simulink model "momentum_dump_test_rev2"  (R2016b)
settings: Solver=VariableStepAuto  StartTime=0.0  StopTime=2500  MinStep=0.001  RelTol=1e-3
values from neighbouring files (symbols this model uses):
  fsw_params = init_fsw_params()    [momentum_unload_test_init.m]
undefined symbols (not defined in the file or in its folder): body_rates_radps, command_processing, DiscIntNeverNeededParam, disturbances_lib, DT_aero_eci_Nm, DT_dipole_body_Am2, DT_grav_eci_Nm, DT_solar_eci_Nm, env_acc_eci_mps2, Environment, environment_lib, GPS_time, init_pos_eci_km, init_vel_eci_kmps, mag_vec_eci, magnetorquer_assembly_lib, position_eci_km, quaternion, RW_assembly_simple_lib, sim_params, sun_vec_eci, velocity_eci_kmps
libraries: aerolibutil x10, simulink x6, bus_stubs_template x3, aerolibactuator x3, vrlib x2, dynamics_lib x1, GPS_time_lib x1, aero_drag_lib x1, gravity_lib_2 x1, mag_vec_lib x1, solar_pressure_lib x1, sun_vector_lib x1
settings Model: Creator=evich  LastModifiedBy=evich

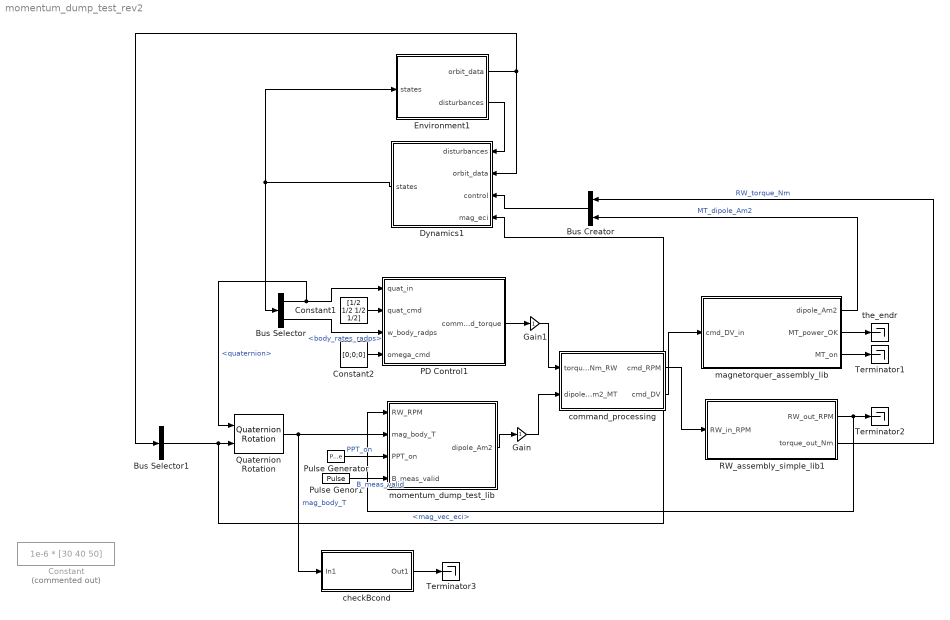
== system momentum_dump_test_rev2 ==
  Bus Creator : BusCreator  Inputs=2
  Bus Selector : BusSelector  OutputSignals=quaternion,body_rates_radps
  Bus Selector1 : BusSelector  OutputSignals=mag_vec_eci
  Constant : Constant  Commented=on  Value=1e-6 * [30 40 50]
  Constant1 : Constant  Value=[1/2 1/2 1/2 1/2]
  Constant2 : Constant  Value=[0;0;0]
  Dynamics1 : Subsystem  AncestorBlock=dynamics_lib/Dynamics
  Environment1 : Subsystem  AncestorBlock=environment_lib/Environment
  Gain : Gain
  Gain1 : Gain
  PD Control1 : Subsystem  AncestorBlock=pd_control_lib/PD Control
  Pulse Generator : DiscretePulseGenerator  PulseType=Time based  Period=fsw_params.actuators.ppt.sync_pulse  PulseWidth=fsw_params.actuators.ppt.t_charge_pct
  Pulse Genor1 : DiscretePulseGenerator  PulseType=Time based  Period=10  PulseWidth=sim_params.sensors.magnetometer.valid_pct
  Quaternion Rotation : aerolibutil/Quaternion Rotation
  RW_assembly_simple_lib1 : Subsystem  AncestorBlock=RW_assembly_simple_lib/RW_assembly_simple_lib  mask{natural_frequency=sim_params.actuators.reaction_wheel.natural_freq, damping_ratio=sim_params.actuators.reaction_wheel.damping, max_rate=sim_params.actuators.reaction_wheel.rate_limit}
      mask prompts: natural_frequency "aeroblks:aeroblkactuator:blockNonlinearSecondOrderActuatorParamNaturalfrequency"; damping_ratio "aeroblks:aeroblkactuator:blockNonlinearSecondOrderActuatorParamDampingratio"; max_rate "aeroblks:aeroblkactuator:blockNonlinearSecondOrderActuatorParamRatelimit"
      mask TypeOptions natural_frequency: Nonlinear Second-Order Actuator/wn_fin | Nonlinear Second-Order Actuator1/wn_fin | Nonlinear Second-Order Actuator2/wn_fin
      mask TypeOptions damping_ratio: Nonlinear Second-Order Actuator/z_fin | Nonlinear Second-Order Actuator1/z_fin | Nonlinear Second-Order Actuator2/z_fin
      mask TypeOptions max_rate: Nonlinear Second-Order Actuator/fin_maxrate | Nonlinear Second-Order Actuator1/fin_maxrate | Nonlinear Second-Order Actuator2/fin_maxrate
  Terminator1 : Terminator
  Terminator2 : Terminator
  Terminator3 : Terminator
  checkBcond : Subsystem
  command_processing : Subsystem  AncestorBlock=command_processing/command_processing
  magnetorquer_assembly_lib : Subsystem  AncestorBlock=magnetorquer_assembly_lib/magnetorquer_assembly_lib
  momentum_dump_test_lib : Subsystem
  the_endr : Terminator
  wires:
  Dynamics1/1(states) -> Environment1/1(states), Bus Selector/1
  Environment1/2(disturbances) -> Dynamics1/1(disturbances)
  Environment1/1(orbit_data) -> Bus Selector1/1, Dynamics1/2(orbit_data)
  Bus Creator/1 -> Dynamics1/3(control)
  RW_assembly_simple_lib1/2(torque_out_Nm) -> Bus Creator/1  "RW_torque_Nm"
  magnetorquer_assembly_lib/1(dipole_Am2) -> Bus Creator/2  "MT_dipole_Am2"
  Bus Selector/1 -> PD Control1/1(quat_in), Quaternion Rotation/1  "<quaternion>"
  Bus Selector/2 -> PD Control1/3(w_body_radps)  "<body_rates_radps>"
  command_processing/1(cmd_RPM) -> RW_assembly_simple_lib1/1(RW_in_RPM)
  command_processing/2(cmd_DV) -> magnetorquer_assembly_lib/1(cmd_DV_in)
  PD Control1/1(command_torque) -> Gain1/1
  momentum_dump_test_lib/1(dipole_Am2) -> Gain/1
  Pulse Generator/1 -> momentum_dump_test_lib/3(PPT_on)  "PPT_on"
  Pulse Genor1/1 -> momentum_dump_test_lib/4(B_meas_valid)  "B_meas_valid"
  Constant1/1 -> PD Control1/2(quat_cmd)
  Constant2/1 -> PD Control1/4(omega_cmd)
  magnetorquer_assembly_lib/2(MT_power_OK) -> the_endr/1
  magnetorquer_assembly_lib/3(MT_on) -> Terminator1/1
  RW_assembly_simple_lib1/1(RW_out_RPM) -> momentum_dump_test_lib/1(RW_RPM), Terminator2/1
  Bus Selector1/1 -> Dynamics1/4(mag_eci), Quaternion Rotation/2  "<mag_vec_eci>"
  Quaternion Rotation/1 -> checkBcond/1(In1), momentum_dump_test_lib/2(mag_body_T)  "mag_body_T"
  Gain/1 -> command_processing/2(dipole_Am2_MT)
  Gain1/1 -> command_processing/1(torque_Nm_RW)
  checkBcond/1(Out1) -> Terminator3/1

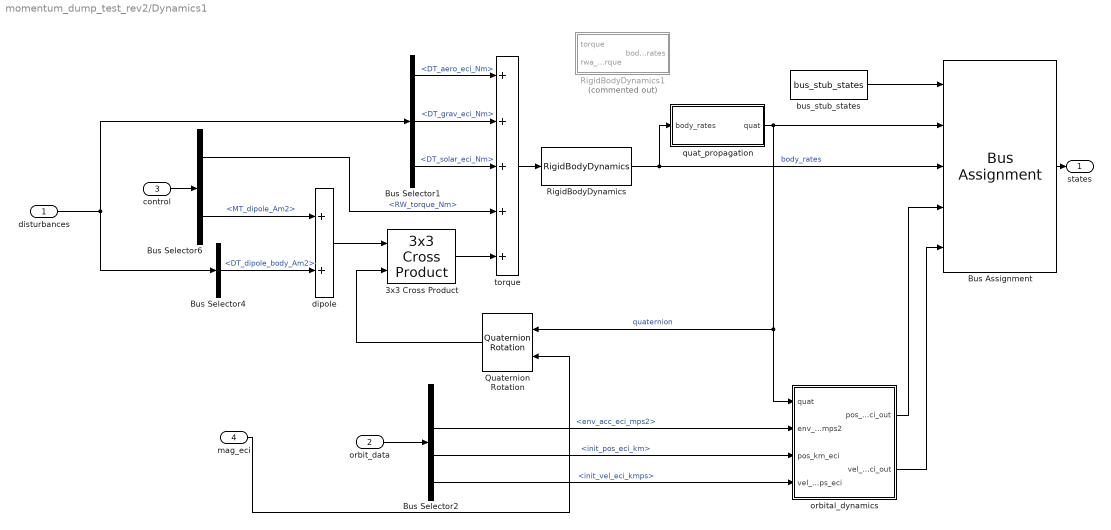
== system momentum_dump_test_rev2/Dynamics1 ==
  disturbances : Inport  OutDataTypeStr=Bus: disturbances
  orbit_data : Inport  Port=2  OutDataTypeStr=Bus: orbit_data
  control : Inport  Port=3  OutDataTypeStr=Bus: control
  mag_eci : Inport  Port=4
  3x3 Cross Product : aerolibutil/3x3 Cross Product
  Bus Assignment : BusAssignment  AssignedSignals=quaternion,body_rates_radps,position_eci_km,velocity_eci_kmps
  Bus Selector1 : BusSelector  OutputSignals=DT_aero_eci_Nm,DT_grav_eci_Nm,DT_solar_eci_Nm
  Bus Selector2 : BusSelector  OutputSignals=mag_vec_eci,env_acc_eci_mps2,init_pos_eci_km,init_vel_eci_kmps
  Bus Selector4 : BusSelector  OutputSignals=DT_dipole_body_Am2
  Bus Selector6 : BusSelector  OutputSignals=RW_torque_Nm,MT_dipole_Am2
  Quaternion Rotation : aerolibutil/Quaternion Rotation
  RigidBodyDynamics : dynamics_lib/Dynamics/RigidBodyDynamics
  RigidBodyDynamics1 : Subsystem  Commented=on
  bus_stub_states : bus_stubs_template/bus_stub_states
  dipole : Sum  Inputs=2
  orbital_dynamics : Subsystem
  quat_propagation : Subsystem
  torque : Sum  Inputs=5
  states : Outport
  wires:
  Bus Assignment/1 -> states/1
  bus_stub_states/1 -> Bus Assignment/1
  quat_propagation/1(quat) -> Bus Assignment/2, Quaternion Rotation/1, orbital_dynamics/1(quat)  "quaternion"
  RigidBodyDynamics/1 -> quat_propagation/1(body_rates), Bus Assignment/3  "body_rates"
  disturbances/1 -> Bus Selector4/1, Bus Selector1/1
  Bus Selector1/1 -> torque/1  "<DT_aero_eci_Nm>"
  Bus Selector1/2 -> torque/2  "<DT_grav_eci_Nm>"
  Bus Selector1/3 -> torque/3  "<DT_solar_eci_Nm>"
  control/1 -> Bus Selector6/1
  Bus Selector6/1 -> torque/4  "<RW_torque_Nm>"
  Bus Selector4/1 -> dipole/2  "<DT_dipole_body_Am2>"
  Bus Selector6/2 -> dipole/1  "<MT_dipole_Am2>"
  torque/1 -> RigidBodyDynamics/1
  dipole/1 -> 3x3 Cross Product/1
  Quaternion Rotation/1 -> 3x3 Cross Product/2
  3x3 Cross Product/1 -> torque/5
  Bus Selector2/2 -> orbital_dynamics/2(env_accel_eci_mps2)  "<env_acc_eci_mps2>"
  mag_eci/1 -> Quaternion Rotation/2
  orbital_dynamics/2(vel_kmps_eci_out) -> Bus Assignment/5
  orbital_dynamics/1(pos_km_eci_out) -> Bus Assignment/4
  Bus Selector2/3 -> orbital_dynamics/3(pos_km_eci)  "<init_pos_eci_km>"
  Bus Selector2/4 -> orbital_dynamics/4(vel_kmps_eci)  "<init_vel_eci_kmps>"
  orbit_data/1 -> Bus Selector2/1

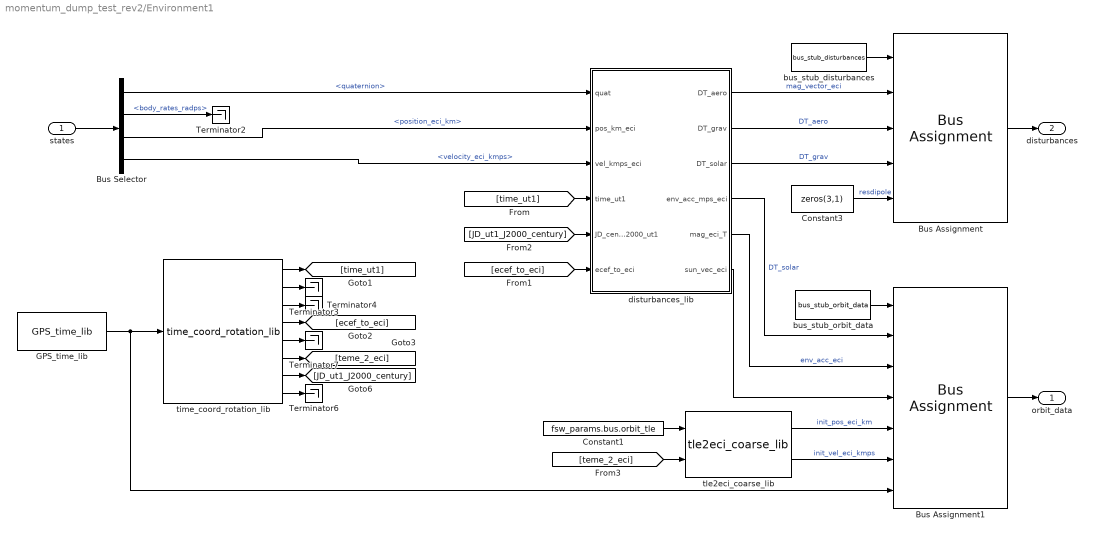
== system momentum_dump_test_rev2/Environment1 ==
  states : Inport  OutDataTypeStr=Bus: states
  Bus Assignment : BusAssignment  AssignedSignals=DT_aero_eci_Nm,DT_grav_eci_Nm,DT_solar_eci_Nm,DT_dipole_body_Am2
  Bus Assignment1 : BusAssignment  AssignedSignals=env_acc_eci_mps2,mag_vec_eci,sun_vec_eci,init_pos_eci_km,init_vel_eci_kmps,GPS_time
  Bus Selector : BusSelector  OutputSignals=quaternion,body_rates_radps,position_eci_km,velocity_eci_kmps
  Constant1 : Constant  Value=fsw_params.bus.orbit_tle
  Constant3 : Constant  Value=zeros(3,1)
  GPS_time_lib : GPS_time_lib/GPS_time_lib
  Terminator{2..4,6..7} (5 alike) : Terminator
  bus_stub_disturbances : bus_stubs_template/bus_stub_disturbances
  bus_stub_orbit_data : bus_stubs_template/bus_stub_orbit_data
  disturbances_lib : Subsystem  AncestorBlock=disturbances_lib/disturbances_lib
  time_coord_rotation_lib : time_coord_rotation_lib/time_coord_rotation_lib
  tle2eci_coarse_lib : tle2eci_coarse_lib/tle2eci_coarse_lib
  orbit_data : Outport
  disturbances : Outport  Port=2
  wires:
  tle2eci_coarse_lib/2 -> Bus Assignment1/6  "init_vel_eci_kmps"
  tle2eci_coarse_lib/1 -> Bus Assignment1/5  "init_pos_eci_km"
  Constant1/1 -> tle2eci_coarse_lib/1
  bus_stub_disturbances/1 -> Bus Assignment/1
  Bus Assignment/1 -> disturbances/1
  states/1 -> Bus Selector/1
  Bus Selector/1 -> disturbances_lib/1(quat)  "<quaternion>"
  Bus Selector/2 -> Terminator2/1  "<body_rates_radps>"
  Bus Selector/3 -> disturbances_lib/2(pos_km_eci)  "<position_eci_km>"
  Bus Selector/4 -> disturbances_lib/3(vel_kmps_eci)  "<velocity_eci_kmps>"
  [time_ut1] -> disturbances_lib/4(time_ut1)
  Constant3/1 -> Bus Assignment/5  "resdipole"
  bus_stub_orbit_data/1 -> Bus Assignment1/1
  Bus Assignment1/1 -> orbit_data/1
  disturbances_lib/6(sun_vec_eci) -> Bus Assignment1/4
  time_coord_rotation_lib/1 -> [time_ut1]
  time_coord_rotation_lib/7 -> [JD_ut1_J2000_century]
  time_coord_rotation_lib/2 -> Terminator3/1
  time_coord_rotation_lib/4 -> [ecef_to_eci]
  [JD_ut1_J2000_century] -> disturbances_lib/5(JD_cent_J2000_ut1)
  [ecef_to_eci] -> disturbances_lib/6(ecef_to_eci)
  disturbances_lib/1(DT_aero) -> Bus Assignment/2  "mag_vector_eci"
  disturbances_lib/2(DT_grav) -> Bus Assignment/3  "DT_aero"
  disturbances_lib/3(DT_solar) -> Bus Assignment/4  "DT_grav"
  disturbances_lib/4(env_acc_mps_eci) -> Bus Assignment1/2  "DT_solar"
  disturbances_lib/5(mag_eci_T) -> Bus Assignment1/3  "env_acc_eci"
  GPS_time_lib/1 -> Bus Assignment1/7, time_coord_rotation_lib/1
  time_coord_rotation_lib/3 -> Terminator4/1
  time_coord_rotation_lib/6 -> [teme_2_eci]
  time_coord_rotation_lib/8 -> Terminator6/1
  time_coord_rotation_lib/5 -> Terminator7/1
  [teme_2_eci] -> tle2eci_coarse_lib/2

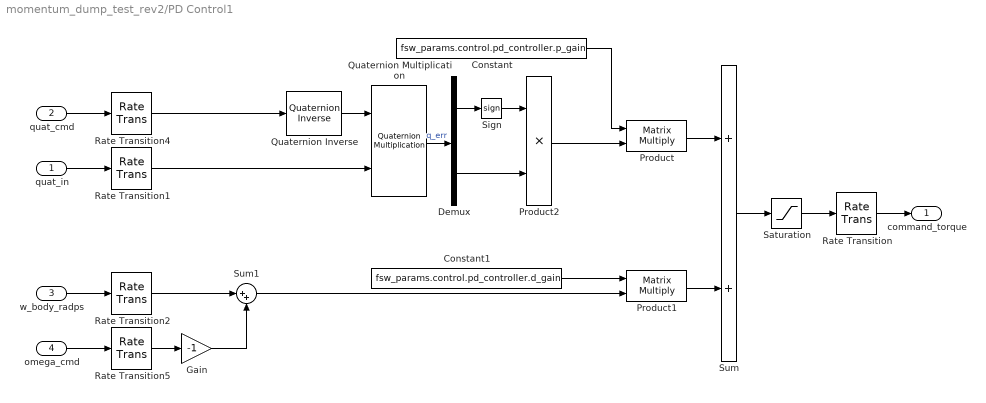
== system momentum_dump_test_rev2/PD Control1 ==
  quat_in : Inport
  quat_cmd : Inport  Port=2
  w_body_radps : Inport  Port=3
  omega_cmd : Inport  Port=4
  Constant : Constant  Value=fsw_params.control.pd_controller.p_gain
  Constant1 : Constant  Value=fsw_params.control.pd_controller.d_gain
  Demux : Demux  Outputs=[1 3]
  Gain : Gain  Gain=-1
  Product : Product  Multiplication=Matrix(*)
  Product1 : Product  Multiplication=Matrix(*)
  Product2 : Product
  Quaternion Inverse : aerolibutil/Quaternion Inverse
  Quaternion Multiplication : aerolibutil/Quaternion Multiplication
  Rate Transition : RateTransition  X0=fsw_params.control.pd_controller.ic.rt_command_torque
  Rate Transition1 : RateTransition  X0=fsw_params.control.pd_controller.ic.rt_quat_in  OutPortSampleTime=fsw_params.control.pd_controller.sample_time_s
  Rate Transition2 : RateTransition  X0=fsw_params.control.pd_controller.ic.rt_w_body_radps  OutPortSampleTime=fsw_params.control.pd_controller.sample_time_s
  Rate Transition4 : RateTransition  X0=fsw_params.control.pd_controller.ic.rt_quat_in  OutPortSampleTime=fsw_params.control.pd_controller.sample_time_s
  Rate Transition5 : RateTransition  X0=fsw_params.control.pd_controller.ic.rt_w_body_radps  OutPortSampleTime=fsw_params.control.pd_controller.sample_time_s
  Saturation : Saturate  UpperLimit=fsw_params.control.pd_controller.max_torque  LowerLimit=-fsw_params.control.pd_controller.max_torque
  Sign : Signum
  Sum : Sum
  Sum1 : Sum  Inputs=|++
  command_torque : Outport
  wires:
  Saturation/1 -> Rate Transition/1
  Constant1/1 -> Product1/1
  Constant/1 -> Product/1
  quat_cmd/1 -> Rate Transition4/1
  Quaternion Inverse/1 -> Quaternion Multiplication/1
  quat_in/1 -> Rate Transition1/1
  Quaternion Multiplication/1 -> Demux/1  "q_err"
  Demux/1 -> Sign/1
  w_body_radps/1 -> Rate Transition2/1
  Demux/2 -> Product2/2
  Product/1 -> Sum/1
  Product1/1 -> Sum/2
  Sum/1 -> Saturation/1
  Rate Transition/1 -> command_torque/1
  Rate Transition1/1 -> Quaternion Multiplication/2
  Rate Transition4/1 -> Quaternion Inverse/1
  omega_cmd/1 -> Rate Transition5/1
  Rate Transition2/1 -> Sum1/1
  Rate Transition5/1 -> Gain/1
  Gain/1 -> Sum1/2
  Sum1/1 -> Product1/2
  Sign/1 -> Product2/1
  Product2/1 -> Product/2

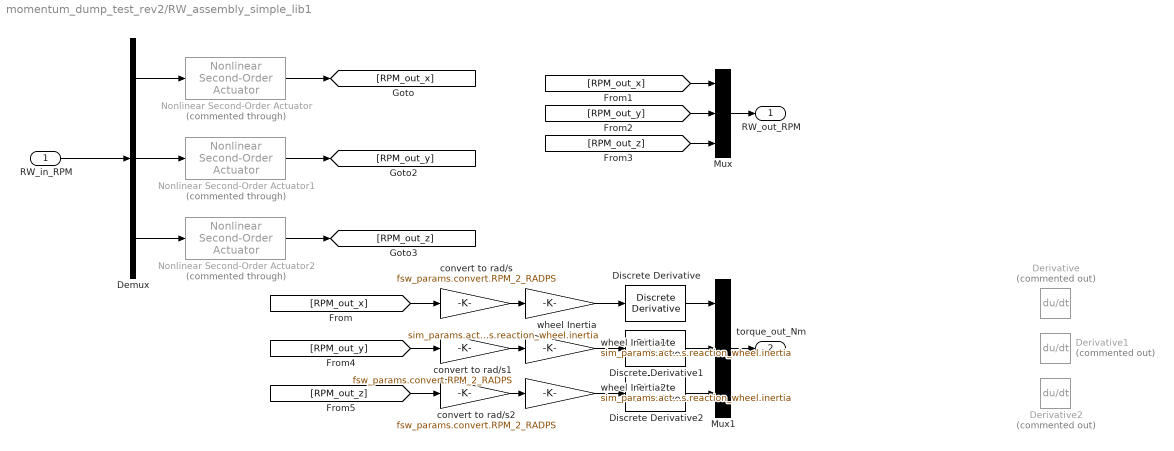
== system momentum_dump_test_rev2/RW_assembly_simple_lib1 ==
  RW_in_RPM : Inport
  Demux : Demux  Outputs=3
  Derivative : Derivative  Commented=on
  Derivative1 : Derivative  Commented=on
  Derivative2 : Derivative  Commented=on
  Discrete Derivative : simulink/Discrete/Discrete Derivative  gainval=1.0  ICPrevScaledInput=sim_params.actuators.reaction_wheel.ic.deriv1  OutMin=[]  OutMax=[]  OutDataType=fixdt(1, 16)  OutScaling=2^-10  DoSatur=off
  Discrete Derivative1 : simulink/Discrete/Discrete Derivative  gainval=1.0  ICPrevScaledInput=sim_params.actuators.reaction_wheel.ic.deriv1  OutMin=[]  OutMax=[]  OutDataType=fixdt(1, 16)  OutScaling=2^-10  DoSatur=off
  Discrete Derivative2 : simulink/Discrete/Discrete Derivative  gainval=1.0  ICPrevScaledInput=sim_params.actuators.reaction_wheel.ic.deriv1  OutMin=[]  OutMax=[]  OutDataType=fixdt(1, 16)  OutScaling=2^-10  DoSatur=off
  Mux : Mux  Inputs=3
  Mux1 : Mux  Inputs=3
  Nonlinear Second-Order Actuator : aerolibactuator/Nonlinear Second-Order Actuator  Commented=through  wn_fin=natural_frequency  z_fin=damping_ratio  fin_max=inf  fin_min=-inf  fin_maxrate=max_rate  fin_act_0=0  fin_act_vel=0
  Nonlinear Second-Order Actuator1 : aerolibactuator/Nonlinear Second-Order Actuator  Commented=through  wn_fin=natural_frequency  z_fin=damping_ratio  fin_max=inf  fin_min=-inf  fin_maxrate=max_rate  fin_act_0=0  fin_act_vel=0
  Nonlinear Second-Order Actuator2 : aerolibactuator/Nonlinear Second-Order Actuator  Commented=through  wn_fin=natural_frequency  z_fin=damping_ratio  fin_max=inf  fin_min=-inf  fin_maxrate=max_rate  fin_act_0=0  fin_act_vel=0
  convert to rad/s : Gain  Gain=fsw_params.convert.RPM_2_RADPS
  convert to rad/s1 : Gain  Gain=fsw_params.convert.RPM_2_RADPS
  convert to rad/s2 : Gain  Gain=fsw_params.convert.RPM_2_RADPS
  wheel Inertia : Gain  Gain=sim_params.actuators.reaction_wheel.inertia
  wheel Inertia1 : Gain  Gain=sim_params.actuators.reaction_wheel.inertia
  wheel Inertia2 : Gain  Gain=sim_params.actuators.reaction_wheel.inertia
  RW_out_RPM : Outport
  torque_out_Nm : Outport  Port=2
  wires:
  RW_in_RPM/1 -> Demux/1
  Demux/1 -> Nonlinear Second-Order Actuator/1
  Demux/2 -> Nonlinear Second-Order Actuator1/1
  Demux/3 -> Nonlinear Second-Order Actuator2/1
  Nonlinear Second-Order Actuator/1 -> [RPM_out_x]
  convert to rad/s/1 -> wheel Inertia/1
  Nonlinear Second-Order Actuator1/1 -> [RPM_out_y]
  Nonlinear Second-Order Actuator2/1 -> [RPM_out_z]
  [RPM_out_x] -> convert to rad/s/1
  [RPM_out_x] -> Mux/1
  [RPM_out_y] -> Mux/2
  [RPM_out_z] -> Mux/3
  Mux/1 -> RW_out_RPM/1
  convert to rad/s1/1 -> wheel Inertia1/1
  [RPM_out_y] -> convert to rad/s1/1
  convert to rad/s2/1 -> wheel Inertia2/1
  [RPM_out_z] -> convert to rad/s2/1
  Mux1/1 -> torque_out_Nm/1
  Discrete Derivative/1 -> Mux1/1
  wheel Inertia/1 -> Discrete Derivative/1
  Discrete Derivative1/1 -> Mux1/2
  Discrete Derivative2/1 -> Mux1/3
  wheel Inertia2/1 -> Discrete Derivative2/1
  wheel Inertia1/1 -> Discrete Derivative1/1

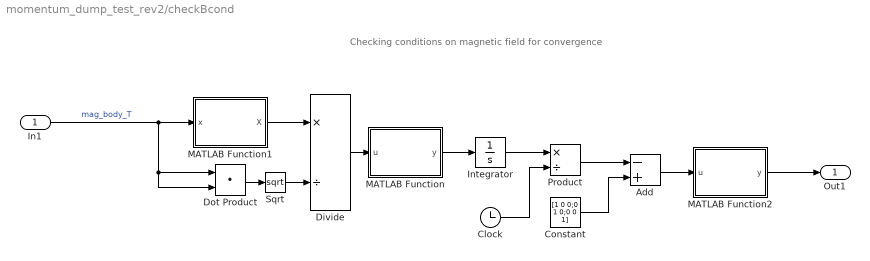
== system momentum_dump_test_rev2/checkBcond ==
  note: Checking conditions on magnetic field for convergence
  In1 : Inport
  Add : Sum  Inputs=-+
  Clock : Clock
      settings: Decimation=10000
  Constant : Constant  Value=[1 0 0;0 1 0;0 0 1]
  Divide : Product  Inputs=*/
  Dot Product : DotProduct  InputSameDT=on  OutDataTypeStr=Inherit: Inherit via internal rule
  Integrator : Integrator  InitialCondition=fsw_params.control.p_dump.ic.delay_B*fsw_params.control.p_dump.ic.delay_B'
  MATLAB Function : MATLAB Function  TreatAsAtomicUnit=on
  MATLAB Function1 : MATLAB Function  TreatAsAtomicUnit=on
  MATLAB Function2 : MATLAB Function  TreatAsAtomicUnit=on
  Product : Product  Inputs=*/
  Sqrt : Sqrt  SaturateOnIntegerOverflow=on
  Out1 : Outport
  wires:
  In1/1 -> Dot Product/2, Dot Product/1, MATLAB Function1/1(x)  "mag_body_T"
  MATLAB Function/1(y) -> Integrator/1
  Integrator/1 -> Product/1
  Clock/1 -> Product/2
  Dot Product/1 -> Sqrt/1
  MATLAB Function1/1(X) -> Divide/1
  Divide/1 -> MATLAB Function/1(u)
  Sqrt/1 -> Divide/2
  Product/1 -> Add/1
  Constant/1 -> Add/2
  Add/1 -> MATLAB Function2/1(u)
  MATLAB Function2/1(y) -> Out1/1

== system momentum_dump_test_rev2/command_processing ==
  torque_Nm_RW : Inport
  dipole_Am2_MT : Inport  Port=2
  dipole-2-digVal : Subsystem
  torque-2-RPM : Subsystem
  cmd_RPM : Outport
  cmd_DV : Outport  Port=2
  wires:
  torque-2-RPM/1(command_RPM) -> cmd_RPM/1
  torque_Nm_RW/1 -> torque-2-RPM/1(cmd_torque_Nm)
  dipole_Am2_MT/1 -> dipole-2-digVal/1(dipole_Am2)
  dipole-2-digVal/1(DigVal) -> cmd_DV/1

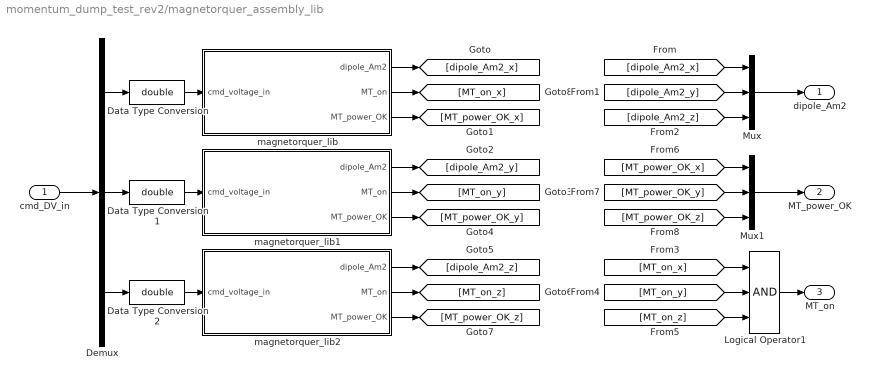
== system momentum_dump_test_rev2/magnetorquer_assembly_lib ==
  cmd_DV_in : Inport
  Data Type Conversion : DataTypeConversion  OutDataTypeStr=double  RndMeth=Nearest
  Data Type Conversion1 : DataTypeConversion  OutDataTypeStr=double  RndMeth=Nearest
  Data Type Conversion2 : DataTypeConversion  OutDataTypeStr=double  RndMeth=Nearest
  Demux : Demux  Outputs=3
  Logical Operator1 : Logic  Inputs=3  AllPortsSameDT=off  OutDataTypeStr=boolean
  Mux : Mux  Inputs=3
  Mux1 : Mux  Inputs=[1 1 1]
  magnetorquer_lib : Subsystem  mask{voltage_to_dipole=fsw_params.control.cmd_processing.dv_2_m_X, upperbound=sim_params.actuators.magnetorquer.max_dipole_x, lowerbound=-sim_params.actuators.magnetorquer.max_dipole_x}
      mask prompts: voltage_to_dipole "Simulink:blkprm_prompts:GainGain"; upperbound "Simulink:masks:UpperBound_MP"; lowerbound "Simulink:masks:LowerBound_MP"
      mask TypeOptions voltage_to_dipole: Gain/Gain
      mask TypeOptions upperbound:
      | Check
      | Static Range/max
      mask TypeOptions lowerbound:
      | Check
      | Static Range/min
  magnetorquer_lib1 : Subsystem  mask{voltage_to_dipole=fsw_params.control.cmd_processing.dv_2_m_Y, upperbound=sim_params.actuators.magnetorquer.max_dipole_y, lowerbound=-sim_params.actuators.magnetorquer.max_dipole_y}
      mask prompts: voltage_to_dipole "Simulink:blkprm_prompts:GainGain"; upperbound "Simulink:masks:UpperBound_MP"; lowerbound "Simulink:masks:LowerBound_MP"
      mask TypeOptions voltage_to_dipole: Gain/Gain
      mask TypeOptions upperbound:
      | Check
      | Static Range/max
      mask TypeOptions lowerbound:
      | Check
      | Static Range/min
  magnetorquer_lib2 : Subsystem  mask{voltage_to_dipole=fsw_params.control.cmd_processing.dv_2_m_Z, upperbound=sim_params.actuators.magnetorquer.max_dipole_z, lowerbound=-sim_params.actuators.magnetorquer.max_dipole_z}
      mask prompts: voltage_to_dipole "Simulink:blkprm_prompts:GainGain"; upperbound "Simulink:masks:UpperBound_MP"; lowerbound "Simulink:masks:LowerBound_MP"
      mask TypeOptions voltage_to_dipole: Gain/Gain
      mask TypeOptions upperbound:
      | Check
      | Static Range/max
      mask TypeOptions lowerbound:
      | Check
      | Static Range/min
  dipole_Am2 : Outport
  MT_power_OK : Outport  Port=2
  MT_on : Outport  Port=3
  wires:
  cmd_DV_in/1 -> Demux/1
  Demux/3 -> Data Type Conversion2/1
  Demux/1 -> Data Type Conversion/1
  Demux/2 -> Data Type Conversion1/1
  magnetorquer_lib/1(dipole_Am2) -> [dipole_Am2_x]
  magnetorquer_lib2/3(MT_power_OK) -> [MT_power_OK_z]
  magnetorquer_lib2/2(MT_on) -> [MT_on_z]
  magnetorquer_lib2/1(dipole_Am2) -> [dipole_Am2_z]
  magnetorquer_lib1/3(MT_power_OK) -> [MT_power_OK_y]
  magnetorquer_lib1/2(MT_on) -> [MT_on_y]
  magnetorquer_lib1/1(dipole_Am2) -> [dipole_Am2_y]
  magnetorquer_lib/3(MT_power_OK) -> [MT_power_OK_x]
  magnetorquer_lib/2(MT_on) -> [MT_on_x]
  Mux/1 -> dipole_Am2/1
  [dipole_Am2_x] -> Mux/1
  [dipole_Am2_y] -> Mux/2
  [dipole_Am2_z] -> Mux/3
  [MT_on_x] -> Logical Operator1/1
  [MT_on_y] -> Logical Operator1/2
  [MT_on_z] -> Logical Operator1/3
  [MT_power_OK_x] -> Mux1/1
  [MT_power_OK_y] -> Mux1/2
  [MT_power_OK_z] -> Mux1/3
  Mux1/1 -> MT_power_OK/1
  Logical Operator1/1 -> MT_on/1
  Data Type Conversion/1 -> magnetorquer_lib/1(cmd_voltage_in)
  Data Type Conversion1/1 -> magnetorquer_lib1/1(cmd_voltage_in)
  Data Type Conversion2/1 -> magnetorquer_lib2/1(cmd_voltage_in)

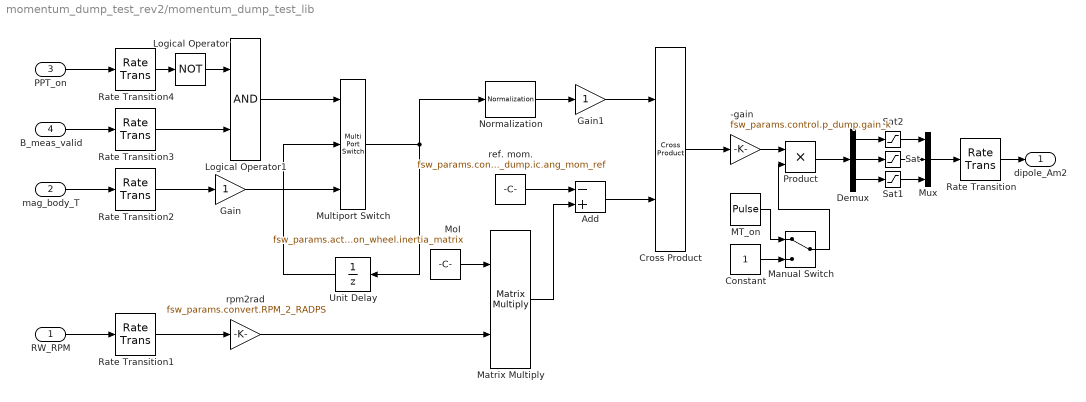
== system momentum_dump_test_rev2/momentum_dump_test_lib ==
  RW_RPM : Inport
  mag_body_T : Inport  Port=2
  PPT_on : Inport  Port=3
  B_meas_valid : Inport  Port=4
  -gain : Gain  Gain=fsw_params.control.p_dump.gain_k
  Add : Sum  Inputs=-+
  Constant : Constant
  Cross Product : vrlib/Utilities/Cross Product
  Demux : Demux  Outputs=3
  Gain : Gain
  Gain1 : Gain
  Logical Operator : Logic  Operator=NOT  AllPortsSameDT=off  OutDataTypeStr=boolean
  Logical Operator1 : Logic  AllPortsSameDT=off  OutDataTypeStr=boolean
  MT_on : DiscretePulseGenerator  PulseType=Time based  Period=1  PulseWidth=fsw_params.actuators.magnetorquer.actuation_time_pct
  Manual Switch : ManualSwitch
  Matrix Multiply : Product  Inputs=**  Multiplication=Matrix(*)
  MoI : Constant  Value=fsw_params.actuators.reaction_wheel.inertia_matrix
  Multiport Switch : MultiPortSwitch  DataPortOrder=Zero-based contiguous  Inputs=2
  Mux : Mux  Inputs=3
  Normalization : dspmathops/Normalization  NormType=Squared 2-norm  Bias=1e-10  NormOver=Each column  Dimension=1  outputDataTypeStr=Inherit: Same as product output  outputLastDataTypeStr=Inherit: Same as product output  outputMin=[]  outputMax=[]  accumDataTypeStr=Inherit: Same as product output  accumLastDataTypeStr=Inherit: Same as product output  roundingMode=Floor  overflowMode=off
  Product : Product
  Rate Transition : RateTransition  X0=fsw_params.control.p_dump.ic.rt_dipole_Am2
  Rate Transition1 : RateTransition  X0=fsw_params.control.p_dump.ic.rt_rw_RPM  OutPortSampleTime=fsw_params.control.p_dump.sample_time_s
  Rate Transition2 : RateTransition  X0=fsw_params.control.p_dump.ic.rt_mag_body_T  OutPortSampleTime=fsw_params.control.p_dump.sample_time_s
  Rate Transition3 : RateTransition  X0=fsw_params.control.p_dump.ic.rt_B_meas_valid  OutPortSampleTime=fsw_params.control.p_dump.sample_time_s
  Rate Transition4 : RateTransition  X0=fsw_params.control.p_dump.ic.rt_PPT_on  OutPortSampleTime=fsw_params.control.p_dump.sample_time_s
  Sat : Saturate  UpperLimit=fsw_params.actuators.magnetorquer.max_dipole_y  LowerLimit=-fsw_params.actuators.magnetorquer.max_dipole_y
  Sat1 : Saturate  UpperLimit=fsw_params.actuators.magnetorquer.max_dipole_z  LowerLimit=-fsw_params.actuators.magnetorquer.max_dipole_z
  Sat2 : Saturate  UpperLimit=fsw_params.actuators.magnetorquer.max_dipole_x  LowerLimit=-fsw_params.actuators.magnetorquer.max_dipole_x
  Unit Delay : UnitDelay  InitialCondition=fsw_params.control.p_dump.ic.rt_mag_body_T  SampleTime=-1
  ref. mom. : Constant  Value=fsw_params.control.p_dump.ic.ang_mom_ref
  rpm2rad : Gain  Gain=fsw_params.convert.RPM_2_RADPS
  dipole_Am2 : Outport
  wires:
  ref. mom./1 -> Add/1
  Matrix Multiply/1 -> Add/2
  MoI/1 -> Matrix Multiply/1
  Multiport Switch/1 -> Normalization/1, Unit Delay/1
  rpm2rad/1 -> Matrix Multiply/2
  Add/1 -> Cross Product/2
  Cross Product/1 -> -gain/1
  Logical Operator1/1 -> Multiport Switch/1
  Logical Operator/1 -> Logical Operator1/1
  Rate Transition3/1 -> Logical Operator1/2
  Rate Transition4/1 -> Logical Operator/1
  Rate Transition2/1 -> Gain/1
  Unit Delay/1 -> Multiport Switch/2
  PPT_on/1 -> Rate Transition4/1
  B_meas_valid/1 -> Rate Transition3/1
  mag_body_T/1 -> Rate Transition2/1
  RW_RPM/1 -> Rate Transition1/1
  Rate Transition1/1 -> rpm2rad/1
  Demux/2 -> Sat/1
  Demux/1 -> Sat2/1
  Demux/3 -> Sat1/1
  Sat1/1 -> Mux/3
  Sat/1 -> Mux/2
  Sat2/1 -> Mux/1
  Mux/1 -> Rate Transition/1
  Gain/1 -> Multiport Switch/3
  Gain1/1 -> Cross Product/1
  Normalization/1 -> Gain1/1
  Rate Transition/1 -> dipole_Am2/1
  -gain/1 -> Product/1
  Product/1 -> Demux/1
  Constant/1 -> Manual Switch/2
  MT_on/1 -> Manual Switch/1
  Manual Switch/1 -> Product/2

== system momentum_dump_test_rev2/Dynamics1/RigidBodyDynamics1 ==
  torque : Inport
  rwa_torque : Inport  Port=2
  Integrator : Integrator  InitialCondition=sim_params.dynamics.ic.rate_init
  Integrator1 : Integrator  InitialCondition=fsw_params.control.cmd_processing.ic.momentum
  dynamics : Subsystem
  body_rates : Outport
  wires:
  dynamics/1(omega_dot) -> Integrator/1
  torque/1 -> dynamics/1(torque)
  Integrator/1 -> dynamics/2(omega), body_rates/1
  rwa_torque/1 -> Integrator1/1
  Integrator1/1 -> dynamics/3(rwa_momentum)

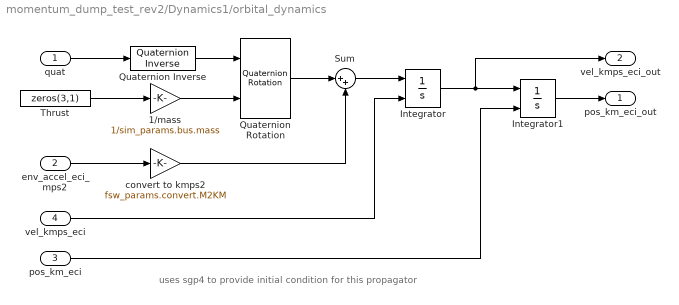
== system momentum_dump_test_rev2/Dynamics1/orbital_dynamics ==
  note: uses sgp4 to provide initial condition for this propagator
  quat : Inport
  env_accel_eci_mps2 : Inport  Port=2
  pos_km_eci : Inport  Port=3
  vel_kmps_eci : Inport  Port=4
  1/mass : Gain  Gain=1/sim_params.bus.mass
  Integrator : Integrator  InitialConditionSource=external  InitialCondition=sim_params.orbit.init_vel_eci
  Integrator1 : Integrator  InitialConditionSource=external  InitialCondition=sim_params.orbit.init_pos_eci
  Quaternion Inverse : aerolibutil/Quaternion Inverse
  Quaternion Rotation : aerolibutil/Quaternion Rotation
  Sum : Sum  Inputs=|++
  Thrust : Constant  Value=zeros(3,1)
  convert to kmps2 : Gain  Gain=fsw_params.convert.M2KM
  pos_km_eci_out : Outport
  vel_kmps_eci_out : Outport  Port=2
  wires:
  convert to kmps2/1 -> Sum/2
  Quaternion Rotation/1 -> Sum/1
  vel_kmps_eci/1 -> Integrator/2
  env_accel_eci_mps2/1 -> convert to kmps2/1
  Integrator/1 -> vel_kmps_eci_out/1, Integrator1/1
  Thrust/1 -> 1/mass/1
  Sum/1 -> Integrator/1
  1/mass/1 -> Quaternion Rotation/2
  Quaternion Inverse/1 -> Quaternion Rotation/1
  pos_km_eci/1 -> Integrator1/2
  quat/1 -> Quaternion Inverse/1
  Integrator1/1 -> pos_km_eci_out/1

== system momentum_dump_test_rev2/Dynamics1/quat_propagation ==
  body_rates : Inport
  Gain1 : Gain  Gain=1/2
  Integrator1 : Integrator  InitialCondition=sim_params.dynamics.ic.quat_init
  MATLAB Function : MATLAB Function  TreatAsAtomicUnit=on
  Product : Product  Multiplication=Matrix(*)  RndMeth=Zero
  Quaternion Normalize : aerolibutil/Quaternion Normalize
  quat : Outport
  wires:
  MATLAB Function/1(Omega) -> Gain1/1
  body_rates/1 -> MATLAB Function/1(w)
  Quaternion Normalize/1 -> Product/2, quat/1
  Gain1/1 -> Product/1
  Integrator1/1 -> Quaternion Normalize/1
  Product/1 -> Integrator1/1

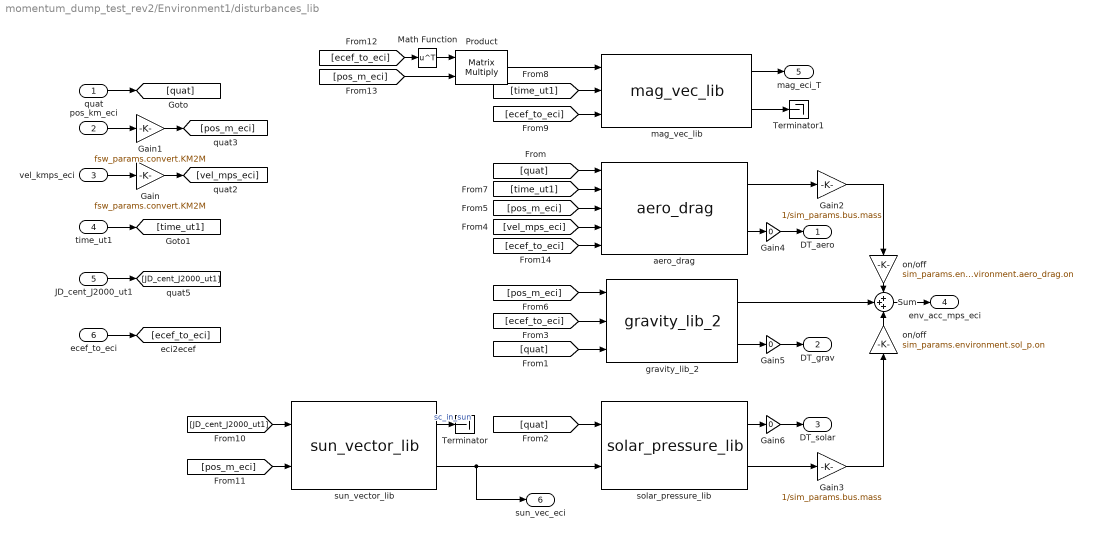
== system momentum_dump_test_rev2/Environment1/disturbances_lib ==
  quat : Inport
  pos_km_eci : Inport  Port=2
  vel_kmps_eci : Inport  Port=3
  time_ut1 : Inport  Port=4
  JD_cent_J2000_ut1 : Inport  Port=5
  ecef_to_eci : Inport  Port=6
  Gain : Gain  Gain=fsw_params.convert.KM2M
  Gain1 : Gain  Gain=fsw_params.convert.KM2M
  Gain2 : Gain  Gain=1/sim_params.bus.mass
  Gain3 : Gain  Gain=1/sim_params.bus.mass
  Gain4 : Gain  Gain=0
  Gain5 : Gain  Gain=0
  Gain6 : Gain  Gain=0
  Math Function : Math  Operator=transpose  SaturateOnIntegerOverflow=on
  Product : Product  Multiplication=Matrix(*)
  Sum : Sum  Inputs=+++
  Terminator : Terminator
  Terminator1 : Terminator
  aero_drag : aero_drag_lib/aero_drag
  gravity_lib_2 : gravity_lib_2/gravity_lib_2
  mag_vec_lib : mag_vec_lib/mag_vec_lib
  on/off : Gain  Gain=sim_params.environment.aero_drag.on
  "on/off " : Gain  Gain=sim_params.environment.sol_p.on
  solar_pressure_lib : solar_pressure_lib/solar_pressure_lib
  sun_vector_lib : sun_vector_lib/sun_vector_lib
  DT_aero : Outport
  DT_grav : Outport  Port=2
  DT_solar : Outport  Port=3
  env_acc_mps_eci : Outport  Port=4
  mag_eci_T : Outport  Port=5
  sun_vec_eci : Outport  Port=6
  wires:
  [ecef_to_eci] -> aero_drag/5
  quat/1 -> [quat]
  ecef_to_eci/1 -> [ecef_to_eci]
  [quat] -> aero_drag/1
  [quat] -> solar_pressure_lib/1
  [ecef_to_eci] -> gravity_lib_2/2
  vel_kmps_eci/1 -> Gain/1
  Gain/1 -> [vel_mps_eci]
  [vel_mps_eci] -> aero_drag/4
  pos_km_eci/1 -> Gain1/1
  Gain1/1 -> [pos_m_eci]
  [pos_m_eci] -> aero_drag/3
  [pos_m_eci] -> gravity_lib_2/1
  time_ut1/1 -> [time_ut1]
  [time_ut1] -> aero_drag/2
  [time_ut1] -> mag_vec_lib/2
  JD_cent_J2000_ut1/1 -> [JD_cent_J2000_ut1]
  [JD_cent_J2000_ut1] -> sun_vector_lib/1
  [pos_m_eci] -> sun_vector_lib/2
  sun_vector_lib/1 -> Terminator/1  "sc_in_sun"
  sun_vector_lib/2 -> sun_vec_eci/1, solar_pressure_lib/2
  [pos_m_eci] -> Product/2
  Product/1 -> mag_vec_lib/1
  mag_vec_lib/2 -> Terminator1/1
  mag_vec_lib/1 -> mag_eci_T/1
  gravity_lib_2/1 -> Sum/2
  aero_drag/1 -> Gain2/1
  Gain2/1 -> on/off/1
  solar_pressure_lib/2 -> Gain3/1
  Gain3/1 -> "on/off "/1
  [ecef_to_eci] -> mag_vec_lib/3
  aero_drag/2 -> Gain4/1
  gravity_lib_2/2 -> Gain5/1
  solar_pressure_lib/1 -> Gain6/1
  Sum/1 -> env_acc_mps_eci/1
  [ecef_to_eci] -> Math Function/1
  Math Function/1 -> Product/1
  on/off/1 -> Sum/1
  "on/off "/1 -> Sum/3
  [quat] -> gravity_lib_2/3
  Gain4/1 -> DT_aero/1
  Gain5/1 -> DT_grav/1
  Gain6/1 -> DT_solar/1

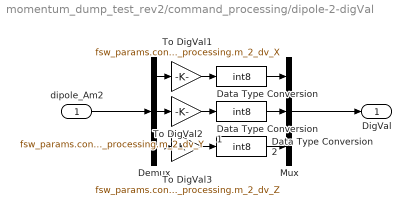
== system momentum_dump_test_rev2/command_processing/dipole-2-digVal ==
  dipole_Am2 : Inport
  Data Type Conversion : DataTypeConversion  OutDataTypeStr=int8  RndMeth=Nearest
  Data Type Conversion1 : DataTypeConversion  OutDataTypeStr=int8  RndMeth=Nearest
  Data Type Conversion2 : DataTypeConversion  OutDataTypeStr=int8  RndMeth=Nearest
  Demux : Demux  Outputs=3
  Mux : Mux  Inputs=3
  To DigVal1 : Gain  Gain=fsw_params.control.cmd_processing.m_2_dv_X
  To DigVal2 : Gain  Gain=fsw_params.control.cmd_processing.m_2_dv_Y
  To DigVal3 : Gain  Gain=fsw_params.control.cmd_processing.m_2_dv_Z
  DigVal : Outport
  wires:
  dipole_Am2/1 -> Demux/1
  Demux/3 -> To DigVal3/1
  Demux/2 -> To DigVal2/1
  Demux/1 -> To DigVal1/1
  To DigVal1/1 -> Data Type Conversion/1
  To DigVal2/1 -> Data Type Conversion1/1
  To DigVal3/1 -> Data Type Conversion2/1
  Mux/1 -> DigVal/1
  Data Type Conversion/1 -> Mux/1
  Data Type Conversion1/1 -> Mux/2
  Data Type Conversion2/1 -> Mux/3

== system momentum_dump_test_rev2/command_processing/torque-2-RPM ==
  cmd_torque_Nm : Inport
  Constant : Constant  Value=fsw_params.actuators.reaction_wheel.inertia_matrix
  Discrete-Time Integrator : DiscreteIntegrator  InitialCondition=fsw_params.control.cmd_processing.ic.momentum  InitialConditionSetting=State (most efficient)  SampleTime=-1  ICPrevOutput=DiscIntNeverNeededParam  ICPrevScaledInput=DiscIntNeverNeededParam
  Integrator : Integrator  Commented=on  InitialCondition=fsw_params.control.cmd_processing.ic.momentum
  Invert 3x3 Matrix : aerolibutil/Invert  3x3 Matrix
  Product : Product  Multiplication=Matrix(*)
  Saturation : Saturate  UpperLimit=fsw_params.actuators.reaction_wheel.max_RPM  LowerLimit=-fsw_params.actuators.reaction_wheel.max_RPM
  radps_2_rpm : Gain  Gain=fsw_params.convert.RADPS_2_RPM
  command_RPM : Outport
  wires:
  Constant/1 -> Invert 3x3 Matrix/1
  Invert 3x3 Matrix/1 -> Product/1
  Product/1 -> radps_2_rpm/1
  radps_2_rpm/1 -> Saturation/1
  cmd_torque_Nm/1 -> Discrete-Time Integrator/1
  Discrete-Time Integrator/1 -> Product/2
  Saturation/1 -> command_RPM/1

== system momentum_dump_test_rev2/magnetorquer_assembly_lib/magnetorquer_lib ==
  cmd_voltage_in : Inport
  Check Static Range : simulink/Model Verification/Check  Static Range  Description=lowerbound <= u <= upperbound  max=upperbound  max_included=on  min=lowerbound  min_included=on  enabled=on  stopWhenAssertionFail=off  export=on  icon=graphic
  Gain : Gain  Gain=voltage_to_dipole
  Pulse Generator : DiscretePulseGenerator  PulseType=Time based  Period=1  PulseWidth=fsw_params.actuators.magnetorquer.actuation_time_pct
  dipole_Am2 : Outport
  MT_on : Outport  Port=2
  MT_power_OK : Outport  Port=3
  wires:
  Check Static Range/1 -> MT_power_OK/1
  Pulse Generator/1 -> MT_on/1
  Gain/1 -> dipole_Am2/1, Check Static Range/1
  cmd_voltage_in/1 -> Gain/1

== system momentum_dump_test_rev2/magnetorquer_assembly_lib/magnetorquer_lib1 ==
  cmd_voltage_in : Inport
  Check Static Range : simulink/Model Verification/Check  Static Range  Description=lowerbound <= u <= upperbound  max=upperbound  max_included=on  min=lowerbound  min_included=on  enabled=on  stopWhenAssertionFail=off  export=on  icon=graphic
  Gain : Gain  Gain=voltage_to_dipole
  Pulse Generator : DiscretePulseGenerator  PulseType=Time based  Period=1  PulseWidth=fsw_params.actuators.magnetorquer.actuation_time_pct
  dipole_Am2 : Outport
  MT_on : Outport  Port=2
  MT_power_OK : Outport  Port=3
  wires:
  Check Static Range/1 -> MT_power_OK/1
  Pulse Generator/1 -> MT_on/1
  Gain/1 -> dipole_Am2/1, Check Static Range/1
  cmd_voltage_in/1 -> Gain/1

== system momentum_dump_test_rev2/magnetorquer_assembly_lib/magnetorquer_lib2 ==
  cmd_voltage_in : Inport
  Check Static Range : simulink/Model Verification/Check  Static Range  Description=lowerbound <= u <= upperbound  max=upperbound  max_included=on  min=lowerbound  min_included=on  enabled=on  stopWhenAssertionFail=off  export=on  icon=graphic
  Gain : Gain  Gain=voltage_to_dipole
  Pulse Generator : DiscretePulseGenerator  PulseType=Time based  Period=1  PulseWidth=fsw_params.actuators.magnetorquer.actuation_time_pct
  dipole_Am2 : Outport
  MT_on : Outport  Port=2
  MT_power_OK : Outport  Port=3
  wires:
  Check Static Range/1 -> MT_power_OK/1
  Pulse Generator/1 -> MT_on/1
  Gain/1 -> dipole_Am2/1, Check Static Range/1
  cmd_voltage_in/1 -> Gain/1

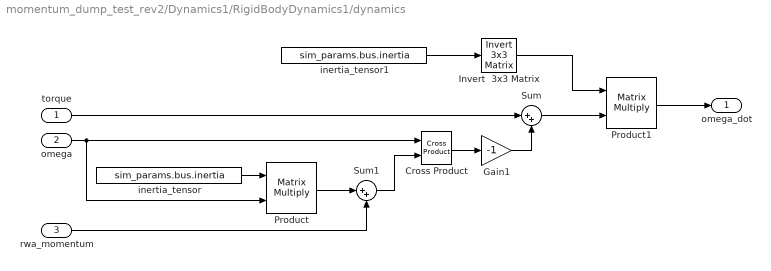
== system momentum_dump_test_rev2/Dynamics1/RigidBodyDynamics1/dynamics ==
  torque : Inport
  omega : Inport  Port=2
  rwa_momentum : Inport  Port=3
  Cross Product : vrlib/Utilities/Cross Product
  Gain1 : Gain  Gain=-1
  Invert  3x3 Matrix : aerolibutil/Invert  3x3 Matrix
  Product : Product  Multiplication=Matrix(*)  RndMeth=Zero
  Product1 : Product  Multiplication=Matrix(*)  RndMeth=Zero
  Sum : Sum  Inputs=|++
  Sum1 : Sum  Inputs=|++
  inertia_tensor : Constant  Value=sim_params.bus.inertia
  inertia_tensor1 : Constant  Value=sim_params.bus.inertia
  omega_dot : Outport
  wires:
  torque/1 -> Sum/1
  omega/1 -> Cross Product/1, Product/2
  inertia_tensor/1 -> Product/1
  Cross Product/1 -> Gain1/1
  Product/1 -> Sum1/1
  Sum/1 -> Product1/2
  Product1/1 -> omega_dot/1
  Invert  3x3 Matrix/1 -> Product1/1
  inertia_tensor1/1 -> Invert  3x3 Matrix/1
  Gain1/1 -> Sum/2
  rwa_momentum/1 -> Sum1/2
  Sum1/1 -> Cross Product/2

== matlab function momentum_dump_test_rev2/Dynamics1/quat_propagation/MATLAB Function ==
  data: w input; Omega output
function Omega = skew_sym(w)
%#codegen

    w_skew = ...
        [0 w(3) -w(2);
        -w(3) 0 w(1);
        w(2) -w(1) 0];

    Omega = ...
        [0 -w';
        w w_skew];

== matlab function momentum_dump_test_rev2/checkBcond/MATLAB Function ==
  data: u input; y output
function y = outerprod(u)

y = u*u';

== matlab function momentum_dump_test_rev2/checkBcond/MATLAB Function1 ==
  data: x input; X output
function X   = skew( x )
% UW HuskySat-1, ADCS Subsystem
% Last Update: E. Hansen 12.8.2017

%Transforms a vector into a skew symmetric matrix (Levi-Civita)
%--------------------------------------------------------------------------

X = [0 -x(3) x(2);x(3) 0 -x(1);-x(2) x(1) 0];

== matlab function momentum_dump_test_rev2/checkBcond/MATLAB Function2 ==
  data: u input; y output
function y = eigval(u)

y = eig(u);
